simulink model "Decode_from_MLC"  (Simulink 8.6)
settings: Solver=VariableStepAuto  StartTime=0.0  StopTime=inf  RelTol=1e-3
libraries: hdlsllib x10, simulink x7
settings Model: Creator=Oscar  LastModifiedBy=Oscar
settings DataIOCC: SaveFormat=Dataset  SignalLoggingSaveFormat=Dataset
settings OptimizationCC: ExpressionDepthLimit=128
settings DebuggingCC: UnderspecifiedInitializationDetection=Simplified  MergeDetectMultiDrivingBlocksExec=error  SolverPrmCheckMsg=none  FcnCallInpInsideContextMsg=EnableAllAsError  StateNameClashWarn=none
settings HardwareCC: ProdBitPerPointer=64  ProdLargestAtomicFloat=Float  ProdIntDivRoundTo=Zero  ProdEndianess=LittleEndian  ProdWordSize=64  ProdHWDeviceType=Intel->x86-64 (Windows64)
settings GRTTargetCC: GeneratePreprocessorConditionals=Use local settings  CombineOutputUpdateFcns=on  GRTInterface=off
settings ConfigComp: CovModelRefEnable=off

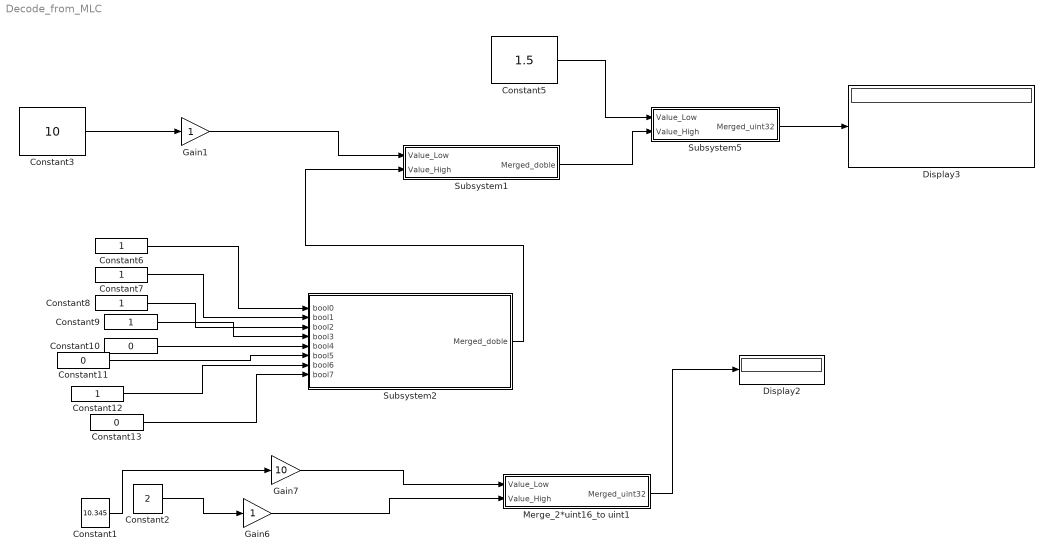
== system Decode_from_MLC ==
  Constant1 : Constant  Value=10.345
  Constant10 : Constant  Value=0
  Constant11 : Constant  Value=0
  Constant{6..9,12} (5 alike) : Constant
  Constant13 : Constant  Value=0
  Constant2 : Constant  Value=2
  Constant3 : Constant  Value=10
  Constant5 : Constant  Value=1.5
  Display2 : Display
  Display3 : Display
      settings: Format=hex (Stored Integer)
  Gain1 : Gain
  Gain6 : Gain
  Gain7 : Gain  Gain=10
  Merge_2*uint16_to uint1 : Subsystem
  Subsystem1 : Subsystem
  Subsystem2 : Subsystem
  Subsystem5 : Subsystem
  wires:
  Constant2/1 -> Gain6/1
  Constant1/1 -> Gain7/1
  Merge_2*uint16_to uint1/1(Merged_uint32) -> Display2/1
  Gain7/1 -> Merge_2*uint16_to uint1/1(Value_Low)
  Gain6/1 -> Merge_2*uint16_to uint1/2(Value_High)
  Constant3/1 -> Gain1/1
  Gain1/1 -> Subsystem1/1(Value_Low)
  Subsystem1/1(Merged_doble) -> Subsystem5/2(Value_High)
  Constant5/1 -> Subsystem5/1(Value_Low)
  Subsystem5/1(Merged_uint32) -> Display3/1
  Constant6/1 -> Subsystem2/1(bool0)
  Constant7/1 -> Subsystem2/2(bool1)
  Constant8/1 -> Subsystem2/3(bool2)
  Constant9/1 -> Subsystem2/4(bool3)
  Constant10/1 -> Subsystem2/5(bool4)
  Constant11/1 -> Subsystem2/6(bool5)
  Constant12/1 -> Subsystem2/7(bool6)
  Constant13/1 -> Subsystem2/8(bool7)
  Subsystem2/1(Merged_doble) -> Subsystem1/2(Value_High)

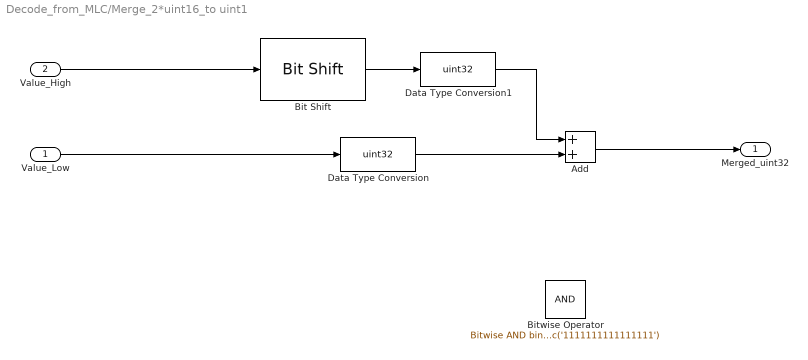
== system Decode_from_MLC/Merge_2*uint16_to uint1 ==
  Value_Low : Inport
  Value_High : Inport  Port=2
  Add : Sum
  Bit Shift : hdlsllib/HDL Operations/Bit Shift  mode=Shift Left Logical  N=16
  Bitwise Operator : simulink/Logic and Bit Operations/Bitwise Operator  logicop=AND  UseBitMask=on  BitMask=bin2dec('1111111111111111')  BitMaskRealWorld=Stored Integer
  Data Type Conversion : DataTypeConversion  OutDataTypeStr=uint32
  Data Type Conversion1 : DataTypeConversion  OutDataTypeStr=uint32
  Merged_uint32 : Outport
  wires:
  Value_Low/1 -> Data Type Conversion/1
  Bit Shift/1 -> Data Type Conversion1/1
  Add/1 -> Merged_uint32/1
  Value_High/1 -> Bit Shift/1
  Data Type Conversion/1 -> Add/2
  Data Type Conversion1/1 -> Add/1

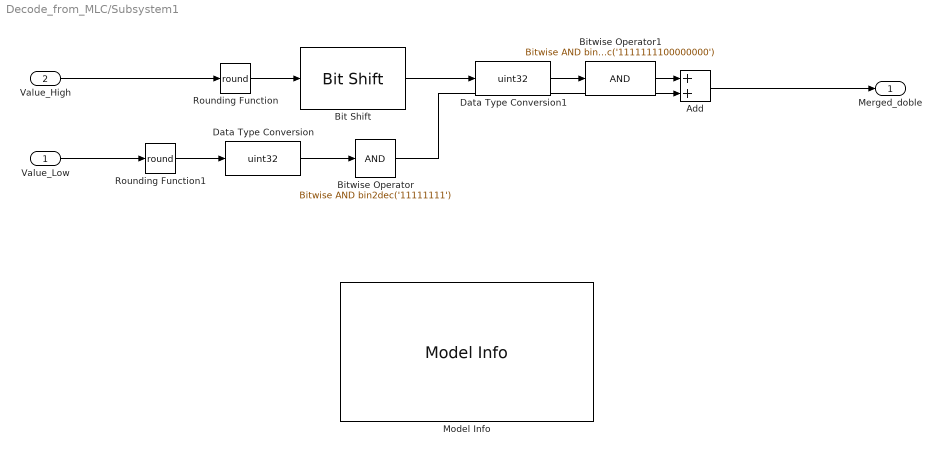
== system Decode_from_MLC/Subsystem1 ==
  Value_Low : Inport
  Value_High : Inport  Port=2
  Add : Sum  OutDataTypeStr=double
  Bit Shift : hdlsllib/HDL Operations/Bit Shift  mode=Shift Left Logical  N=8
  Bitwise Operator : simulink/Logic and Bit Operations/Bitwise Operator  logicop=AND  UseBitMask=on  BitMask=bin2dec('11111111')  BitMaskRealWorld=Stored Integer
  Bitwise Operator1 : simulink/Logic and Bit Operations/Bitwise Operator  logicop=AND  UseBitMask=on  BitMask=bin2dec('1111111100000000')  BitMaskRealWorld=Stored Integer
  Data Type Conversion : DataTypeConversion  OutDataTypeStr=uint32
  Data Type Conversion1 : DataTypeConversion  OutDataTypeStr=uint32
  Model Info : simulink/Model-Wide Utilities/Model Info  Frame=on  DisplayStringWithTags=|  HorizontalTextAlignment=Center  LeftAlignmentValue=0.5  SourceBlockDiagram=Decode_from_MLC  TagMaxNumber=20
      | %<Created>
      | %<Creator>
      | 
      | Shift and round two double values into one double value.
      | 
      | input:	two double values (treated as 8-bit)
      | output:	One double value(treated as 16-bit)
  Rounding Function : Rounding  Operator=round
  Rounding Function1 : Rounding  Operator=round
  Merged_doble : Outport
  wires:
  Bit Shift/1 -> Data Type Conversion1/1
  Data Type Conversion1/1 -> Bitwise Operator1/1
  Rounding Function/1 -> Bit Shift/1
  Data Type Conversion/1 -> Bitwise Operator/1
  Bitwise Operator/1 -> Add/2
  Rounding Function1/1 -> Data Type Conversion/1
  Bitwise Operator1/1 -> Add/1
  Add/1 -> Merged_doble/1
  Value_Low/1 -> Rounding Function1/1
  Value_High/1 -> Rounding Function/1

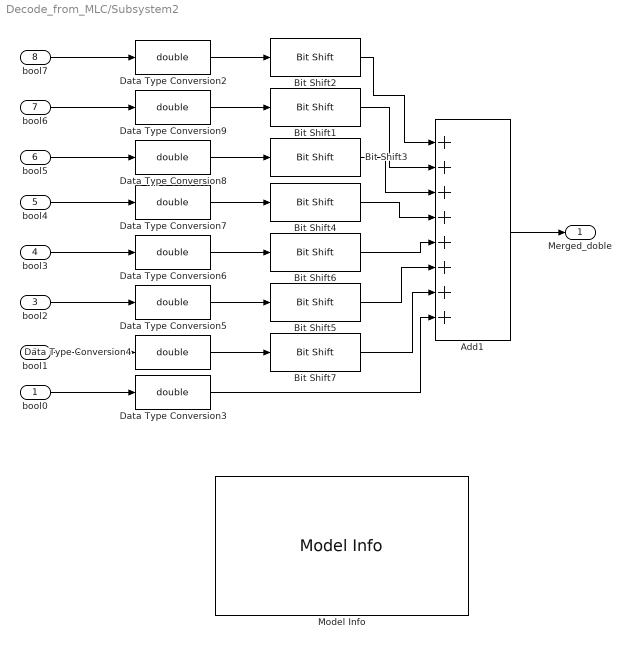
== system Decode_from_MLC/Subsystem2 ==
  bool0 : Inport
  bool1 : Inport  Port=2
  bool2 : Inport  Port=3
  bool3 : Inport  Port=4
  bool4 : Inport  Port=5
  bool5 : Inport  Port=6
  bool6 : Inport  Port=7
  bool7 : Inport  Port=8
  Add1 : Sum  Inputs=++++++++  OutDataTypeStr=double
  Bit Shift1 : hdlsllib/HDL Operations/Bit Shift  mode=Shift Left Logical  N=6
  Bit Shift2 : hdlsllib/HDL Operations/Bit Shift  mode=Shift Left Logical  N=7
  Bit Shift3 : hdlsllib/HDL Operations/Bit Shift  mode=Shift Left Logical  N=5
  Bit Shift4 : hdlsllib/HDL Operations/Bit Shift  mode=Shift Left Logical  N=4
  Bit Shift5 : hdlsllib/HDL Operations/Bit Shift  mode=Shift Left Logical  N=2
  Bit Shift6 : hdlsllib/HDL Operations/Bit Shift  mode=Shift Left Logical  N=3
  Bit Shift7 : hdlsllib/HDL Operations/Bit Shift  mode=Shift Left Logical  N=1
  Data Type Conversion{2..9} (8 alike) : DataTypeConversion  OutDataTypeStr=double
  Model Info : simulink/Model-Wide Utilities/Model Info  Frame=on  DisplayStringWithTags=|  HorizontalTextAlignment=Center  LeftAlignmentValue=0.5  SourceBlockDiagram=Decode_from_MLC  TagMaxNumber=20
      | %<Created>
      | %<Creator>
      | 
      | Shift and round eight double values into one double value.
      | 
      | input:	Eight boolean values
      | output:	One double value(treated as 8-bit)
  Merged_doble : Outport
  wires:
  bool7/1 -> Data Type Conversion2/1
  Data Type Conversion2/1 -> Bit Shift2/1
  Bit Shift2/1 -> Add1/1
  Bit Shift1/1 -> Add1/2
  Bit Shift3/1 -> Add1/3
  Bit Shift4/1 -> Add1/4
  Bit Shift6/1 -> Add1/5
  Bit Shift5/1 -> Add1/6
  Bit Shift7/1 -> Add1/7
  Data Type Conversion3/1 -> Add1/8
  bool0/1 -> Data Type Conversion3/1
  Data Type Conversion4/1 -> Bit Shift7/1
  Data Type Conversion9/1 -> Bit Shift1/1
  Data Type Conversion8/1 -> Bit Shift3/1
  Data Type Conversion7/1 -> Bit Shift4/1
  Data Type Conversion6/1 -> Bit Shift6/1
  Data Type Conversion5/1 -> Bit Shift5/1
  bool1/1 -> Data Type Conversion4/1
  bool2/1 -> Data Type Conversion5/1
  bool3/1 -> Data Type Conversion6/1
  bool4/1 -> Data Type Conversion7/1
  bool5/1 -> Data Type Conversion8/1
  bool6/1 -> Data Type Conversion9/1
  Add1/1 -> Merged_doble/1

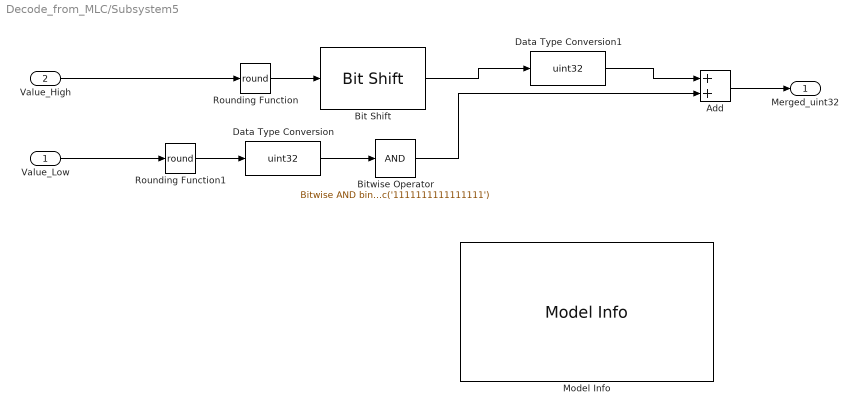
== system Decode_from_MLC/Subsystem5 ==
  Value_Low : Inport
  Value_High : Inport  Port=2
  Add : Sum
  Bit Shift : hdlsllib/HDL Operations/Bit Shift  mode=Shift Left Logical  N=16
  Bitwise Operator : simulink/Logic and Bit Operations/Bitwise Operator  logicop=AND  UseBitMask=on  BitMask=bin2dec('1111111111111111')  BitMaskRealWorld=Stored Integer
  Data Type Conversion : DataTypeConversion  OutDataTypeStr=uint32
  Data Type Conversion1 : DataTypeConversion  OutDataTypeStr=uint32
  Model Info : simulink/Model-Wide Utilities/Model Info  Frame=on  DisplayStringWithTags=|  HorizontalTextAlignment=Center  LeftAlignmentValue=0.5  SourceBlockDiagram=Decode_from_MLC  TagMaxNumber=20
      | %<Created>
      | %<Creator>
      | 
      | Shift and round two double values into one double value.
      | 
      | input:	two double values (treated as 16-bit)
      | output:	One uint32 value
  Rounding Function : Rounding  Operator=round
  Rounding Function1 : Rounding  Operator=round
  Merged_uint32 : Outport
  wires:
  Bit Shift/1 -> Data Type Conversion1/1
  Data Type Conversion1/1 -> Add/1
  Rounding Function/1 -> Bit Shift/1
  Data Type Conversion/1 -> Bitwise Operator/1
  Add/1 -> Merged_uint32/1
  Bitwise Operator/1 -> Add/2
  Rounding Function1/1 -> Data Type Conversion/1
  Value_High/1 -> Rounding Function/1
  Value_Low/1 -> Rounding Function1/1
